simulink model "BFSK"  (R2018a)
settings: Solver=VariableStepAuto  StartTime=0.0  StopTime=10.0  RelTol=1e-3
libraries: dspmathops x2, dspsrcs4 x2, commsynccomp2 x1, commrandsrc3 x1, commutil2 x1, commanapbnd3 x1, simulink_extras x1, dspfdesign x1
settings Model: Creator=Subhankar  LastModifiedBy=Souhardhya Paul

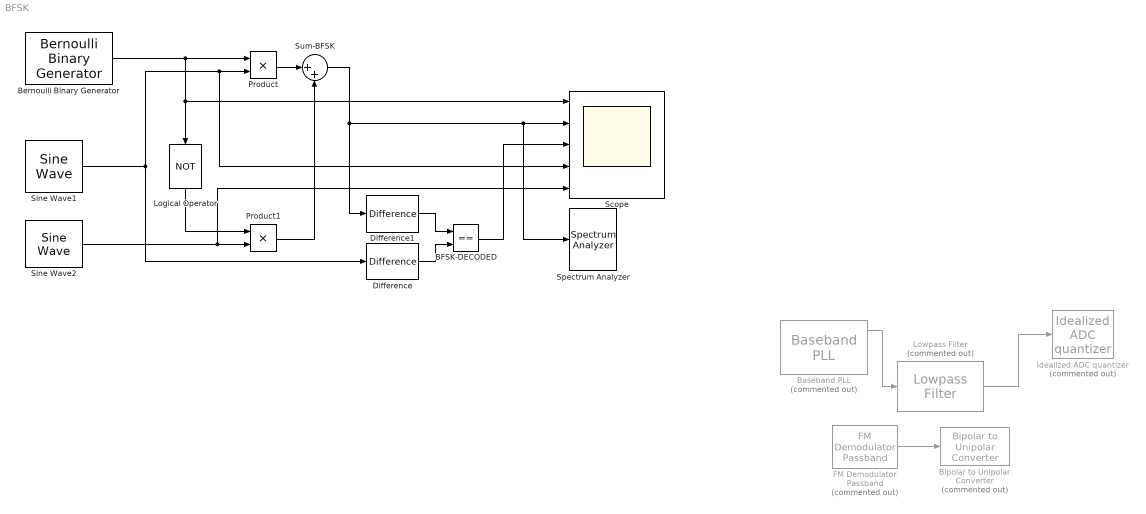
== system BFSK ==
  BFSK-DECODED : RelationalOperator  Operator===  OutDataTypeStr=boolean  RndMeth=Simplest
  Baseband PLL : commsynccomp2/Baseband PLL  Commented=on  Fn="[3.0002  0  40002]"  Fd="[1   67.46   2270.9   40002]"  Kvco=1
      settings: SourceProductName=Communications System Toolbox  SourceProductBaseCode=CM
  Bernoulli Binary Generator : commrandsrc3/Bernoulli Binary Generator  ProbabilityOfZero=0.5  SeedSource=Parameter  Seed=61  SampleTime=0.1  SamplesPerFrame=1  OutputDataType=double  SimulateUsing=Interpreted execution
  Bipolar to Unipolar Converter : commutil2/Bipolar to Unipolar Converter  Commented=on  M=2  polarity=Positive  dataType=Inherit via internal rule
      settings: SourceProductName=Communications System Toolbox  SourceProductBaseCode=CM
  Difference : dspmathops/Difference  Run=Yes  dim=Columns  Dimension=1  roundingMode=Floor  overflowMode=off  outputDataTypeStr=Inherit: Same as accumulator  outputMin=[]  outputMax=[]  outputLastDataTypeStr=Inherit: Same as accumulator
      settings: SourceProductName=DSP System Toolbox  SourceProductBaseCode=DS
  Difference1 : dspmathops/Difference  Run=Yes  dim=Columns  Dimension=1  roundingMode=Floor  overflowMode=off  outputDataTypeStr=Inherit: Same as accumulator  outputMin=[]  outputMax=[]  outputLastDataTypeStr=Inherit: Same as accumulator
      settings: SourceProductName=DSP System Toolbox  SourceProductBaseCode=DS
  FM Demodulator Passband : commanapbnd3/FM Demodulator Passband  Commented=on  Fc=150  Ph=0  Kc=150  Ho=100
      settings: SourceProductName=Communications System Toolbox  SourceProductBaseCode=CM
  Idealized ADC quantizer : simulink_extras/Additional Discrete/Idealized ADC quantizer  Commented=on  NumberOfConverterBits=12  Vmin=0  Vmax=5  OutputDataType=int16  OutputNegativeValues=off
      settings: SourceProductName=Simulink
  Logical Operator : Logic  Operator=NOT  AllPortsSameDT=off  OutDataTypeStr=boolean
  Lowpass Filter : dspfdesign/Lowpass Filter  Commented=on  FilterType=FIR  DesignForMinimumOrder=on  FilterOrder=50  PassbandFrequency=10  StopbandFrequency=80  PassbandRipple=1  StopbandAttenuation=60  InheritSampleRate=on  SampleRate=100  SimulateUsing=Interpreted execution  roundingMode=Floor  coeffsDataTypeStr=fixdt(1,16)
  Product : Product
  Product1 : Product
  Scope : Scope  NumInputPorts=5
  Sine Wave1 : dspsrcs4/Sine Wave  Amplitude=1  Frequency=200  Phase=0  SampleMode=Discrete  OutComplex=Real  CompMethod=Trigonometric fcn  TableSize=Speed  SampleTime=1/1000  SamplesPerFrame=1  ResetState=Restart at time zero  OutputFrames=off  dataType=double  wordLen=16  udDataType=sfix(16)  fracBitsMode=Best precision  numFracBits=15  OutDataTypeStr=double  LastOutDataTypeStr=double
  Sine Wave2 : dspsrcs4/Sine Wave  Amplitude=1  Frequency=100  Phase=0  SampleMode=Discrete  OutComplex=Real  CompMethod=Trigonometric fcn  TableSize=Speed  SampleTime=1/1000  SamplesPerFrame=1  ResetState=Restart at time zero  OutputFrames=off  dataType=double  wordLen=16  udDataType=sfix(16)  fracBitsMode=Best precision  numFracBits=15  OutDataTypeStr=double  LastOutDataTypeStr=double
  Spectrum Analyzer : SpectrumAnalyzer
  Sum-BFSK : Sum  Inputs=|++
  wires:
  Bernoulli Binary Generator/1 -> Product/1, Scope/1, Logical Operator/1
  Logical Operator/1 -> Product1/1
  Sine Wave2/1 -> Product1/2, Scope/5
  Sine Wave1/1 -> Product/2, Scope/4, Difference/1
  Product/1 -> Sum-BFSK/1
  Product1/1 -> Sum-BFSK/2
  Sum-BFSK/1 -> Scope/2, Spectrum Analyzer/1, Difference1/1
  Baseband PLL/1 -> Lowpass Filter/1
  Lowpass Filter/1 -> Idealized ADC quantizer/1
  FM Demodulator Passband/1 -> Bipolar to Unipolar Converter/1
  Difference1/1 -> BFSK-DECODED/1
  Difference/1 -> BFSK-DECODED/2
  BFSK-DECODED/1 -> Scope/3
